simulink model "msdDoubleBuilding"  (R2020b)
settings: Solver=VariableStepAuto  StartTime=0.0  StopTime=150  MaxStep=0.01  RelTol=1e-6
settings Model: Creator=Rocksmithed  LastModifiedBy=Rocksmithed
settings DataIOCC: SaveFormat=Array

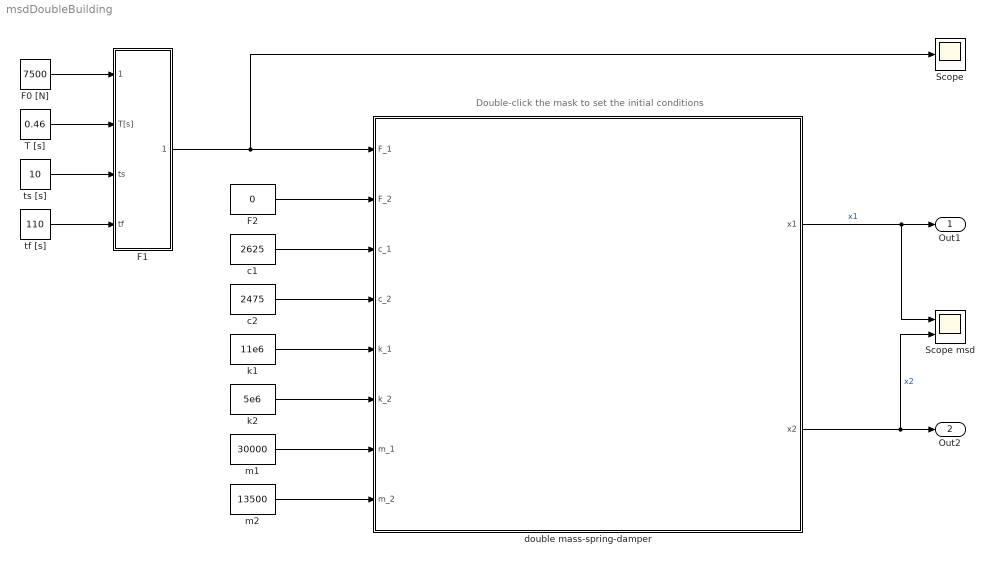
== system msdDoubleBuilding ==
  note: Double-click the mask to set the initial conditions
  F0 [N] : Constant  Value=7500
  F1 : Subsystem
  F2 : Constant  Value=0
  Scope : Scope
  Scope msd : Scope  NumInputPorts=2
  T [s] : Constant  Value=0.46
  c1 : Constant  Value=2625
  c2 : Constant  Value=2475
  double mass-spring-damper : Subsystem  mask{x1_0=0, x2_0=0, x1_dot_0=0, x2_dot_0=0}
      mask prompts: x1_0 "x1(0)"; x2_0 "x2(0)"; x1_dot_0 "x1_dot(0)"; x2_dot_0 "x2_dot(0)"
      mask Display: image('$imagefile'); % Use "Edit Image" on toolstrip to change.
  k1 : Constant  Value=11e6
  k2 : Constant  Value=5e6
  m1 : Constant  Value=30000
  m2 : Constant  Value=13500
  tf [s] : Constant  Value=110
  ts [s] : Constant  Value=10
  Out1 : Outport
  Out2 : Outport  Port=2
  wires:
  F1/1(Out1) -> double mass-spring-damper/1(F_1), Scope/1
  T [s]/1 -> F1/2(T[s])
  F0 [N]/1 -> F1/1(F0 [N])
  F2/1 -> double mass-spring-damper/2(F_2)
  c1/1 -> double mass-spring-damper/3(c_1)
  c2/1 -> double mass-spring-damper/4(c_2)
  k1/1 -> double mass-spring-damper/5(k_1)
  k2/1 -> double mass-spring-damper/6(k_2)
  m1/1 -> double mass-spring-damper/7(m_1)
  m2/1 -> double mass-spring-damper/8(m_2)
  double mass-spring-damper/1(x1) -> Scope msd/1, Out1/1  "x1"
  double mass-spring-damper/2(x2) -> Scope msd/2, Out2/1  "x2"
  ts [s]/1 -> F1/3(ts)
  tf [s]/1 -> F1/4(tf)

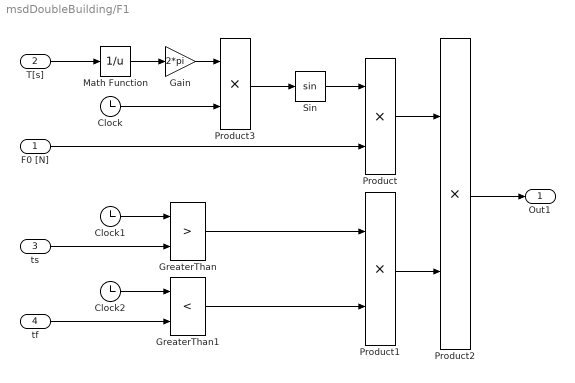
== system msdDoubleBuilding/F1 ==
  F0 [N] : Inport
  T[s] : Inport  Port=2
  ts : Inport  Port=3
  tf : Inport  Port=4
  Clock : Clock
  Clock1 : Clock
  Clock2 : Clock
  Gain : Gain  Gain=2*pi
  GreaterThan : RelationalOperator  Operator=>  OutDataTypeStr=boolean  RndMeth=Simplest
  GreaterThan1 : RelationalOperator  Operator=<  OutDataTypeStr=boolean  RndMeth=Simplest
  Math Function : Math  Operator=reciprocal  SaturateOnIntegerOverflow=on
  Product{,1..3} (4 alike) : Product
  Sin : Trigonometry
  Out1 : Outport
  wires:
  GreaterThan/1 -> Product1/1
  GreaterThan1/1 -> Product1/2
  Product2/1 -> Out1/1
  Product/1 -> Product2/1
  Product1/1 -> Product2/2
  Math Function/1 -> Gain/1
  Gain/1 -> Product3/1
  Clock/1 -> Product3/2
  Product3/1 -> Sin/1
  Sin/1 -> Product/1
  F0 [N]/1 -> Product/2
  T[s]/1 -> Math Function/1
  Clock1/1 -> GreaterThan/1
  ts/1 -> GreaterThan/2
  Clock2/1 -> GreaterThan1/1
  tf/1 -> GreaterThan1/2

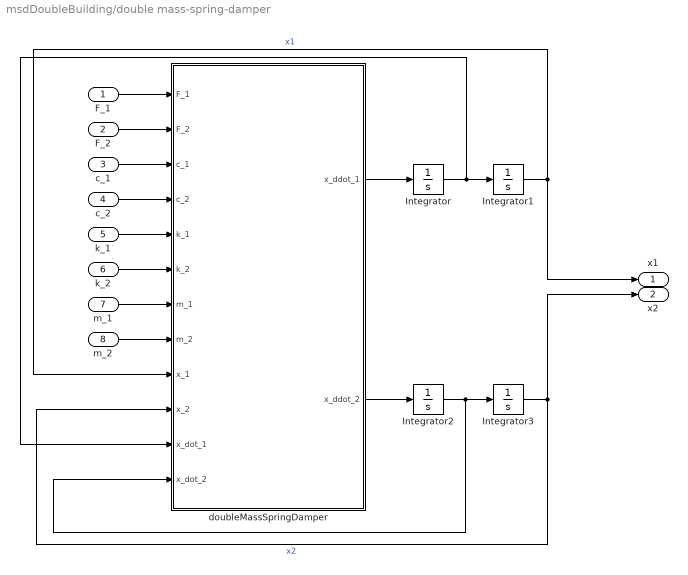
== system msdDoubleBuilding/double mass-spring-damper ==
  F_1 : Inport
  F_2 : Inport  Port=2
  c_1 : Inport  Port=3
  c_2 : Inport  Port=4
  k_1 : Inport  Port=5
  k_2 : Inport  Port=6
  m_1 : Inport  Port=7
  m_2 : Inport  Port=8
  Integrator : Integrator  InitialCondition=x1_dot_0
  Integrator1 : Integrator  InitialCondition=x1_0
  Integrator2 : Integrator  InitialCondition=x2_dot_0
  Integrator3 : Integrator  InitialCondition=x2_0
  doubleMassSpringDamper : MATLAB Function  TreatAsAtomicUnit=on
  x1 : Outport
  x2 : Outport  Port=2
  wires:
  doubleMassSpringDamper/2(x_ddot_2) -> Integrator2/1
  doubleMassSpringDamper/1(x_ddot_1) -> Integrator/1
  k_2/1 -> doubleMassSpringDamper/6(k_2)
  m_2/1 -> doubleMassSpringDamper/8(m_2)
  Integrator/1 -> doubleMassSpringDamper/11(x_dot_1), Integrator1/1
  Integrator1/1 -> x1/1, doubleMassSpringDamper/9(x_1)  "x1"
  Integrator3/1 -> x2/1, doubleMassSpringDamper/10(x_2)  "x2"
  m_1/1 -> doubleMassSpringDamper/7(m_1)
  c_1/1 -> doubleMassSpringDamper/3(c_1)
  Integrator2/1 -> doubleMassSpringDamper/12(x_dot_2), Integrator3/1
  F_1/1 -> doubleMassSpringDamper/1(F_1)
  k_1/1 -> doubleMassSpringDamper/5(k_1)
  F_2/1 -> doubleMassSpringDamper/2(F_2)
  c_2/1 -> doubleMassSpringDamper/4(c_2)

== matlab function msdDoubleBuilding/double mass-spring-damper/doubleMassSpringDamper ==
  data: F_1 input; x_ddot_1 output; F_2 input; c_1 input; c_2 input; k_1 input; k_2 input; m_1 input; m_2 input; x_1 input; x_2 input; x_dot_1 input; x_dot_2 input; x_ddot_2 output
function [x_ddot_1,x_ddot_2] = doubleMassSpringDamper(F_1,F_2,c_1,c_2,k_1,k_2,m_1,m_2,x_1,x_2,x_dot_1,x_dot_2)
%#codegen

%    This function was generated by the Symbolic Math Toolbox version 8.6.
%    19-Nov-2020 15:46:02

x_ddot_1 = -(-F_1+c_1.*x_dot_1+k_1.*x_1+c_2.*(x_dot_1-x_dot_2)+k_2.*(x_1-x_2))./m_1;
if nargout > 1
    x_ddot_2 = (F_2+c_2.*(x_dot_1-x_dot_2)+k_2.*(x_1-x_2))./m_2;
end
